simulink model "Traditional_SMC"  (R2019b)
settings: Solver=VariableStepAuto  StartTime=0.0  StopTime=100  RelTol=1e-3
settings Model: Creator=Asus  LastModifiedBy=Asus

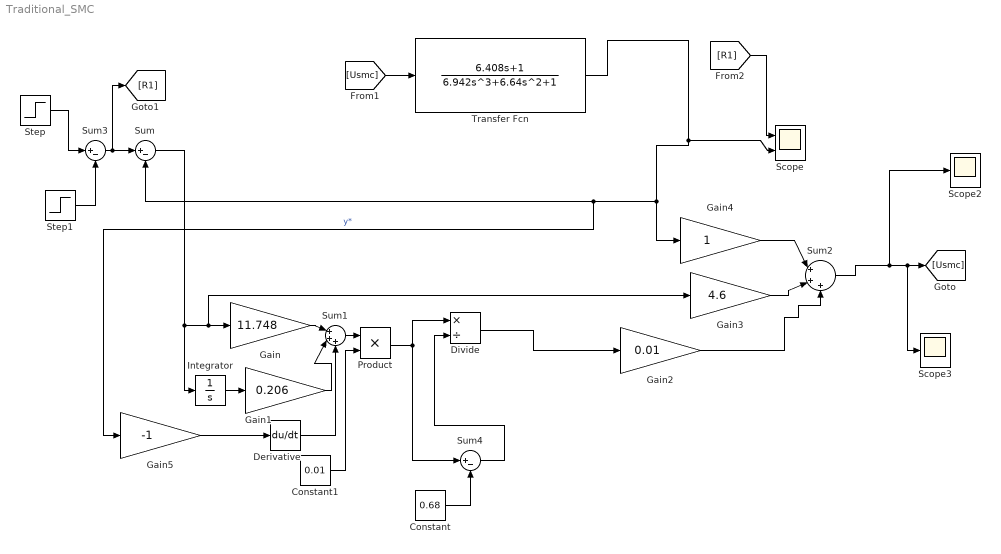
== system Traditional_SMC ==
  Constant : Constant  Value=0.68
  Constant1 : Constant  Value=0.01
  Derivative : Derivative
  Divide : Product  Inputs=*/
  Gain : Gain  Gain=11.748
  Gain1 : Gain  Gain=0.206
  Gain2 : Gain  Gain=0.01
  Gain3 : Gain  Gain=4.6
  Gain4 : Gain
  Gain5 : Gain  Gain=-1
  Integrator : Integrator
  Product : Product
  Scope : Scope  NumInputPorts=2
  Scope2 : Scope
  Scope3 : Scope
  Step : Step  Time=5  SampleTime=0
  Step1 : Step  Time=60  After=0.5  SampleTime=0
  Sum : Sum  Inputs=|+-
  Sum1 : Sum  Inputs=|+++
  Sum2 : Sum  Inputs=|+++
  Sum3 : Sum  Inputs=|+-
  Sum4 : Sum  Inputs=|+-
  Transfer Fcn : TransferFcn  Numerator=[6.408 1]  Denominator=[6.942 6.64 0 1]
  wires:
  Step/1 -> Sum3/1
  Gain1/1 -> Sum1/2
  Sum1/1 -> Product/1
  Product/1 -> Divide/1, Sum4/1
  Constant/1 -> Sum4/2
  Divide/1 -> Gain2/1
  Constant1/1 -> Product/2
  Gain2/1 -> Sum2/3
  Step1/1 -> Sum3/2
  Gain5/1 -> Derivative/1
  Sum3/1 -> [R1], Sum/1
  Sum4/1 -> Divide/2
  [Usmc] -> Transfer Fcn/1
  [R1] -> Scope/1
  Gain/1 -> Sum1/1
  Transfer Fcn/1 -> Gain5/1, Sum/2, Gain4/1, Scope/2  "y*"
  Gain4/1 -> Sum2/1
  Gain3/1 -> Sum2/2
  Derivative/1 -> Sum1/3
  Sum/1 -> Gain3/1, Gain/1, Integrator/1
  Integrator/1 -> Gain1/1
  Sum2/1 -> Scope2/1, Scope3/1, [Usmc]
